simulink model "TwoLinkRobotCL_OpFb"  (R2018b)
settings: Solver=VariableStepAuto  StartTime=0.0  StopTime=5  RelTol=1e-3
values from neighbouring files (symbols this model uses):
  DeltaSim =     [RandomDelta.mat]    (also in twoLinkRobot_BuildLTVModel.m = ss(0,0,0,0))
  xhat0 = [0;0;0;0]    [twoLinkRobot_BuildLTVModel.m]    (also in twoLinkRobot_BuildLTVModel.mat = [0 0 0 0]; twoLinkRobot_HinfDesign.m; twoLinkRobot_HinfDesign.mat = [0 0 0 0])
libraries: ltvlib x7, simulink x1
settings Model: Creator=pjseiler  LastModifiedBy=Jyot Buch
settings SFSimCC: SimUseLocalCustomCode=off
settings RTWCC: RTWUseLocalCustomCode=off
settings CodeAppCC: StateflowObjectComments=on

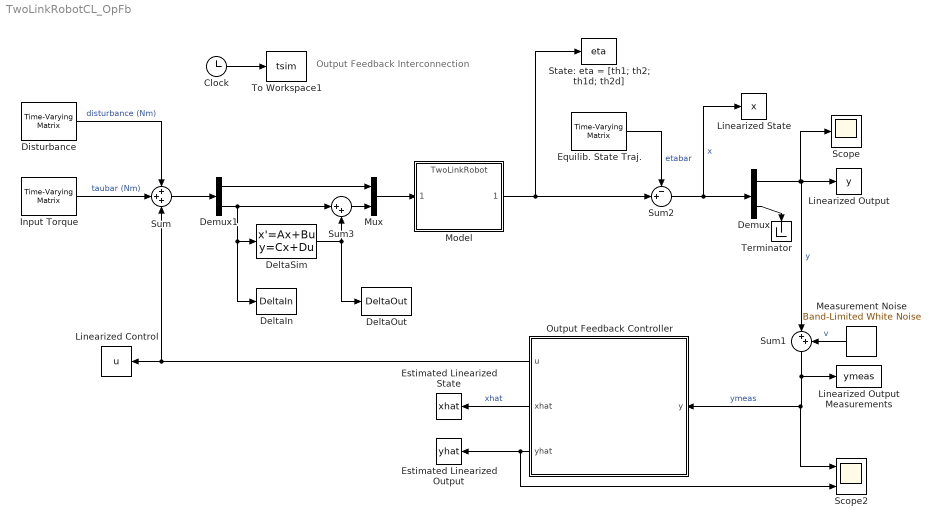
== system TwoLinkRobotCL_OpFb ==
  note: Output Feedback Interconnection
  Clock : Clock
  DeltaIn : ToWorkspace  VariableName=DeltaIn  SampleTime=-1
  DeltaOut : ToWorkspace  VariableName=DeltaOut  SampleTime=-1
  DeltaSim : StateSpace  A=DeltaSim.A  B=DeltaSim.B  C=DeltaSim.C  D=DeltaSim.D  InitialCondition=0
  Demux : Demux  Outputs=[2,2]
  Demux1 : Demux  Outputs=2
  Disturbance : ltvlib/Time-Varying Matrix  M=d  vec1D=on
      settings: SourceProductName=Linear Time-Varying Systems Toolbox
  Equilib. State Traj. : ltvlib/Time-Varying Matrix  M=etabar  vec1D=on
      settings: SourceProductName=Linear Time-Varying Systems Toolbox
  Estimated Linearized Output : ToWorkspace  VariableName=yhat  SampleTime=-1
  Estimated Linearized State : ToWorkspace  VariableName=xhat  SampleTime=-1
  Input Torque : ltvlib/Time-Varying Matrix  M=taubar  vec1D=on
      settings: SourceProductName=Linear Time-Varying Systems Toolbox
  Linearized Control : ToWorkspace  VariableName=u  SampleTime=-1
  Linearized Output : ToWorkspace  VariableName=y  SampleTime=-1
  Linearized Output Measurements : ToWorkspace  VariableName=ymeas  SampleTime=-1
  Linearized State : ToWorkspace  VariableName=x  SampleTime=-1
  Measurement Noise : simulink/Sources/Band-Limited White Noise  Cov=NoisePowerSim  Ts=0.001  seed=[23341,23341]
  Model : ModelReference  ModelNameDialog=TwoLinkRobot.slx  SimulationMode=Normal  ModelReferenceVersion=1.4
  Mux : Mux  Inputs=2
  Output Feedback Controller : Subsystem
  Scope : Scope
  Scope2 : Scope  NumInputPorts=2
  State: eta = [th1; th2; th1d; th2d] : ToWorkspace  VariableName=eta  SampleTime=-1
  Sum : Sum  Inputs=+++
  Sum1 : Sum  Inputs=|++
  Sum2 : Sum  Inputs=-+|
  Sum3 : Sum  Inputs=|++
  Terminator : Terminator
  To Workspace1 : ToWorkspace  VariableName=tsim  SampleTime=-1
  wires:
  Clock/1 -> To Workspace1/1
  Disturbance/1 -> Sum/1  "disturbance (Nm)"
  Model/1 -> State: eta = [th1; th2; th1d; th2d]/1, Sum2/2
  Equilib. State Traj./1 -> Sum2/1  "etabar"
  Sum2/1 -> Linearized State/1, Demux/1  "x"
  Input Torque/1 -> Sum/2  "taubar (Nm)"
  Demux/1 -> Linearized Output/1, Sum1/1, Scope/1  "y"
  Measurement Noise/1 -> Sum1/2  "v"
  Output Feedback Controller/2(xhat) -> Estimated Linearized State/1  "xhat"
  Demux/2 -> Terminator/1
  Output Feedback Controller/1(u) -> Sum/3, Linearized Control/1
  Sum1/1 -> Linearized Output Measurements/1, Scope2/1, Output Feedback Controller/1(y)  "ymeas"
  Output Feedback Controller/3(yhat) -> Estimated Linearized Output/1, Scope2/2
  Demux1/1 -> Mux/1
  Sum3/1 -> Mux/2
  Sum/1 -> Demux1/1
  Demux1/2 -> Sum3/1, DeltaIn/1, DeltaSim/1
  DeltaSim/1 -> DeltaOut/1, Sum3/2
  Mux/1 -> Model/1

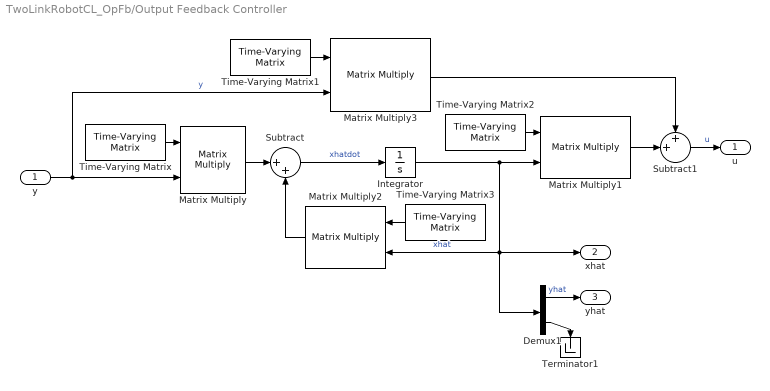
== system TwoLinkRobotCL_OpFb/Output Feedback Controller ==
  y : Inport
  Demux1 : Demux  Outputs=[2,2]
  Integrator : Integrator  InitialCondition=xhat0
  Matrix Multiply{,1..3} (4 alike) : Product  Multiplication=Matrix(*)
  Subtract : Sum  Inputs=|++
  Subtract1 : Sum  Inputs=++|
  Terminator1 : Terminator
  Time-Varying Matrix : ltvlib/Time-Varying Matrix  M=KOpFb.B  vec1D=on
      settings: SourceProductName=Linear Time-Varying Systems Toolbox
  Time-Varying Matrix1 : ltvlib/Time-Varying Matrix  M=KOpFb.D  vec1D=on
      settings: SourceProductName=Linear Time-Varying Systems Toolbox
  Time-Varying Matrix2 : ltvlib/Time-Varying Matrix  M=KOpFb.C  vec1D=on
      settings: SourceProductName=Linear Time-Varying Systems Toolbox
  Time-Varying Matrix3 : ltvlib/Time-Varying Matrix  M=KOpFb.A  vec1D=on
      settings: SourceProductName=Linear Time-Varying Systems Toolbox
  u : Outport
  xhat : Outport  Port=2
  yhat : Outport  Port=3
  wires:
  Matrix Multiply2/1 -> Subtract/2
  y/1 -> Matrix Multiply3/2, Matrix Multiply/2  "y"
  Time-Varying Matrix1/1 -> Matrix Multiply3/1
  Time-Varying Matrix/1 -> Matrix Multiply/1
  Time-Varying Matrix3/1 -> Matrix Multiply2/1
  Matrix Multiply/1 -> Subtract/1
  Matrix Multiply3/1 -> Subtract1/1
  Subtract/1 -> Integrator/1  "xhatdot"
  Matrix Multiply1/1 -> Subtract1/2
  Time-Varying Matrix2/1 -> Matrix Multiply1/1
  Subtract1/1 -> u/1  "u"
  Demux1/1 -> yhat/1  "yhat"
  Integrator/1 -> Matrix Multiply1/2, Demux1/1, Matrix Multiply2/2, xhat/1  "xhat"
  Demux1/2 -> Terminator1/1
